simulink model "ess_adapt_cs"  (Simulink 4.00)
settings: Solver=ode1  SolverMode=SingleTasking  StartTime=0.0  StopTime=29  FixedStep=1  RelTol=1e-3
undefined symbols (not defined in the file or in its folder): ess_soc_current, EssAdaptTime, EssReqAdaptPwr
libraries: lib_energy_storage x1
settings Model: LastModifiedBy=bjeanner  UnconnectedOutputMsg=none

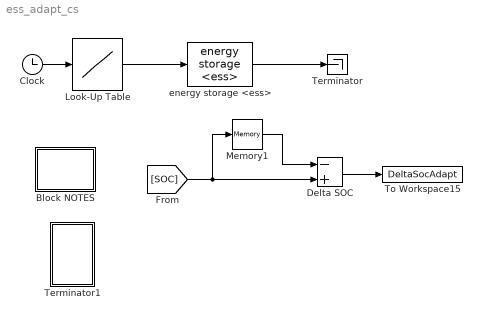
== system ess_adapt_cs ==
  Block NOTES : Subsystem
      settings: RTWFcnNameOpts=Auto  RTWFileNameOpts=Auto
      mask Display: disp('Block\nNOTES')
  Clock : Clock
  Delta SOC : Sum  Inputs=-+  SaturateOnIntegerOverflow=on
  Look-Up Table : Lookup  InputValues=EssAdaptTime  OutputValues=EssReqAdaptPwr
  Memory1 : Memory  X0=ess_soc_current  InheritSampleTime=off
      settings: RTWStateStorageClass=Auto
  Terminator : Terminator
  Terminator1 : Subsystem
      settings: RTWFcnNameOpts=Auto  RTWFileNameOpts=Auto
  To Workspace15 : ToWorkspace  VariableName=DeltaSocAdapt  SampleTime=-1  SaveFormat=Array
  energy storage <ess> : lib_energy_storage/energy storage <ess>  AncestorBlock=lib_energy_storage/Subsystem/energy storage <ess>
      link override ess config: BlockChoice=energy storage <ess>
  wires:
  Look-Up Table/1 -> energy storage <ess>/1
  energy storage <ess>/1 -> Terminator/1
  [SOC] -> Delta SOC/2, Memory1/1
  Memory1/1 -> Delta SOC/1
  Delta SOC/1 -> To Workspace15/1
  Clock/1 -> Look-Up Table/1

== system ess_adapt_cs/Block NOTES ==
  note: This block diagram runs with the fuel cell adaptive control strategy.
      | It is called by the sfun_fuelcell_adapt.m script.
      |
      | Input:
      | Power required from the energy storage (assign in the sfunction)
      | Temperature the energy storage (assign in the sfunction)
      | SOC the energy storage (assign in the sfunction)
      | Output:
      | Delta Soc over one time step (1 sec.)

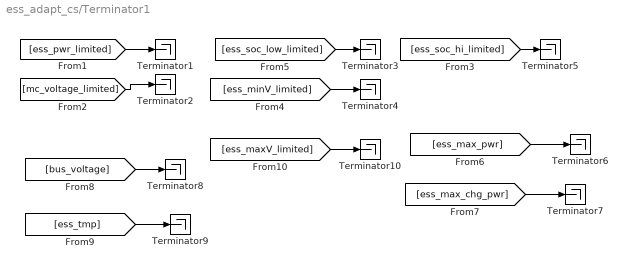
== system ess_adapt_cs/Terminator1 ==
  Terminator{1..10} (10 alike) : Terminator
  wires:
  [ess_pwr_limited] -> Terminator1/1
  [mc_voltage_limited] -> Terminator2/1
  [ess_soc_low_limited] -> Terminator3/1
  [ess_minV_limited] -> Terminator4/1
  [ess_soc_hi_limited] -> Terminator5/1
  [ess_max_pwr] -> Terminator6/1
  [ess_max_chg_pwr] -> Terminator7/1
  [bus_voltage] -> Terminator8/1
  [ess_tmp] -> Terminator9/1
  [ess_maxV_limited] -> Terminator10/1
